simulink model "Task5_without_Scalar"  (R2023b)
settings: Solver=FixedStepAuto  StartTime=0.0  StopTime=300  FixedStep=.02  RelTol=1e-3
InitFcn:
  | run("Longitudinal_Autopilot.m")
values from neighbouring files (symbols this model uses):
  A_Long = [Xu                    Xw                        -w0                            -gravity*cos(theta0) ... (first row only)    [Longitudinal_Autopilot.m]
  B_Long = [Xde                         Xdth ... (first row only)    [Longitudinal_Autopilot.m]
  C_Long = eye(4)    [Longitudinal_Autopilot.m]
  D_Long = zeros(4,2)    [Longitudinal_Autopilot.m]
undefined symbols (not defined in the file or in its folder): sigbuilder_block, states_0, theta0, u0, w0
libraries: simulink_extras x28, cstblocks x21, slpidlib x5
settings Model: Creator=Saif Mohamed  LastModifiedBy=Saif Mohamed

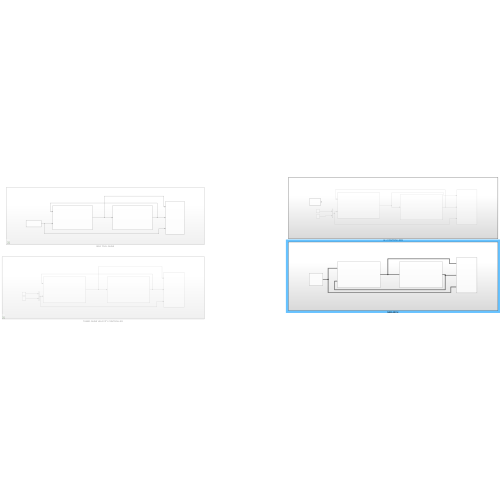
[thumbnail: Simulink's stored preview of the top-level diagram]
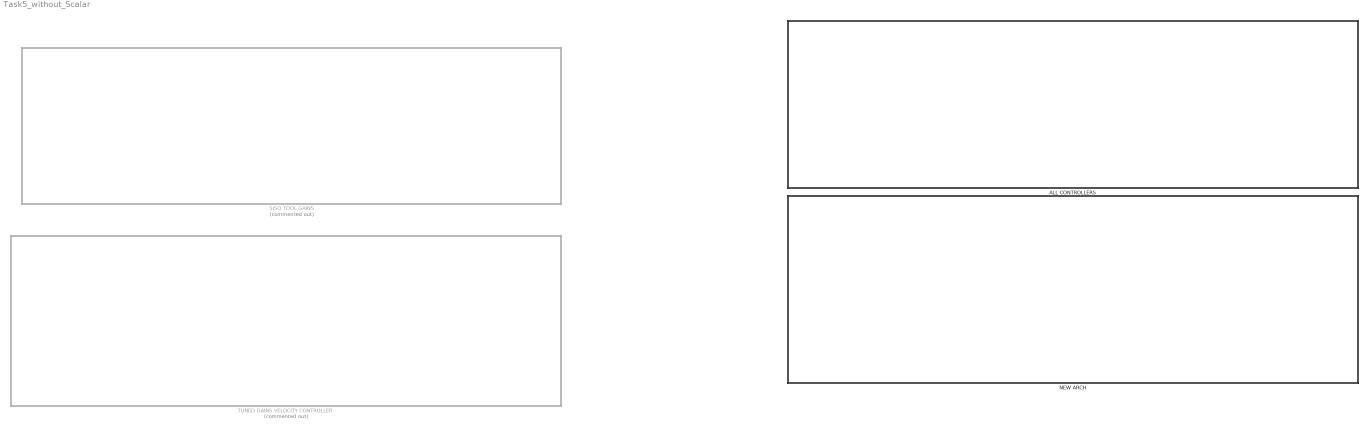
== system Task5_without_Scalar ==
  ALL CONTROLLERS : Subsystem
  "NEW ARCH " : Subsystem
  SISO TOOL GAINS : Subsystem  Commented=on
  "TUNED GAINS VELOCITY CONTROLLER " : Subsystem  Commented=on

== system Task5_without_Scalar/ALL CONTROLLERS ==
  Bus Creator1 : BusCreator  Commented=on  Inputs=2
  Constant2 : Constant  Commented=on  Value=100
  Constant3 : Constant  Commented=on  Value=20
  Display1 : Subsystem  Commented=on
  Longitudinal Model with height : Subsystem  Commented=on
  Signal Builder : Subsystem  Tag=STV Subsys  Commented=on  LoadFcn=sigbuilder_block('load');  StartFcn=sigbuilder_block('start');  StopFcn=sigbuilder_block('stop');  ClipboardFcn=sigbuilder_block('clipboard');  mask(Sigbuilder block){tuvar=[0:10]}
      mask help: Simulink:masks:SigbuilderBlock_MD
      mask init:
      | if ~strcmp(get_param(bdroot(gcbh),'SimulationStatus'),'stopped') tuvar = sigbuilder_block('maskInit'); end
      settings: CopyFcn=sigbuilder_block('copy');  DeleteFcn=sigbuilder_block('delete');  ModelCloseFcn=sigbuilder_block('modelClose');  PreSaveFcn=sigbuilder_block('preSave');  PauseFcn=sigbuilder_block('pause');  ContinueFcn=sigbuilder_block('continue');  NameChangeFcn=sigbuilder_block('namechange');  OpenFcn=sigbuilder_block('open',[5.4 36 1141.2 516.6 ]);  CloseFcn=sigbuilder_block('close');
      mask Display: plot(0, 0, 100, 100,[2, 2, 32, 32, 2], [68, 8, 8, 68, 68],[32, 2], [38, 38], [32, 19, 2],[53, 60, 44], [32, 17, 17, 2],[16, 16, 31, 31]);txt = getActiveGroup(gcbh);text(2, 100, txt,'verticalAlignment', 'top');
  State Space Model1 : Subsystem  Commented=on
  wires:
  Constant2/1 -> Bus Creator1/1  "height_comm"
  Longitudinal Model with height/1(Control_Actions) -> State Space Model1/1(Control_Actions), Display1/1(Control_Actions)
  Constant3/1 -> Bus Creator1/2  "u_command"
  State Space Model1/1(deltas) -> Display1/2(deltas), Longitudinal Model with height/1(deltas)
  Bus Creator1/1 -> Longitudinal Model with height/2(Command), Display1/3(Command)

== system Task5_without_Scalar/NEW ARCH  ==
  Display2 : Subsystem
  Longitudinal Model1 : Subsystem
  State Space Model2 : Subsystem
  Subsystem : Subsystem
  wires:
  Longitudinal Model1/1(Control_Actions) -> Display2/1(Control_Actions), State Space Model2/1(Control_Actions)
  Subsystem/1(Commands) -> Longitudinal Model1/1(Commands), Display2/3(Commands)
  State Space Model2/1(states) -> Longitudinal Model1/2(states), Display2/2(states)

== system Task5_without_Scalar/SISO TOOL GAINS ==
  Display3 : Subsystem
  Longitudinal Model2 : Subsystem
  State Space Model3 : Subsystem
  Subsystem : Subsystem
  wires:
  Longitudinal Model2/1(Control_Actions) -> Display3/1(Control_Actions), State Space Model3/1(Control_Actions)
  State Space Model3/1(deltas) -> Longitudinal Model2/1(deltas), Display3/2(deltas)
  Subsystem/1(Commands) -> Display3/3(Command), Longitudinal Model2/2(Commands)

== system Task5_without_Scalar/TUNED GAINS VELOCITY CONTROLLER  ==
  Bus Creator : BusCreator  Commented=on  Inputs=2
  Constant : Constant  Commented=on
  Constant1 : Constant  Commented=on  Value=10
  Display : Subsystem  Commented=on
  Longitudinal Model : Subsystem  Commented=on
  State Space Model : Subsystem  Commented=on
  wires:
  State Space Model/1(deltas) -> Longitudinal Model/1(deltas), Display/2(deltas)
  Longitudinal Model/1(Control_Actions) -> Display/1(Control_Actions), State Space Model/1(Control_Actions)
  Bus Creator/1 -> Display/3(Command), Longitudinal Model/2(Command)
  Constant/1 -> Bus Creator/1  "theta_command"
  Constant1/1 -> Bus Creator/2  "u_command"

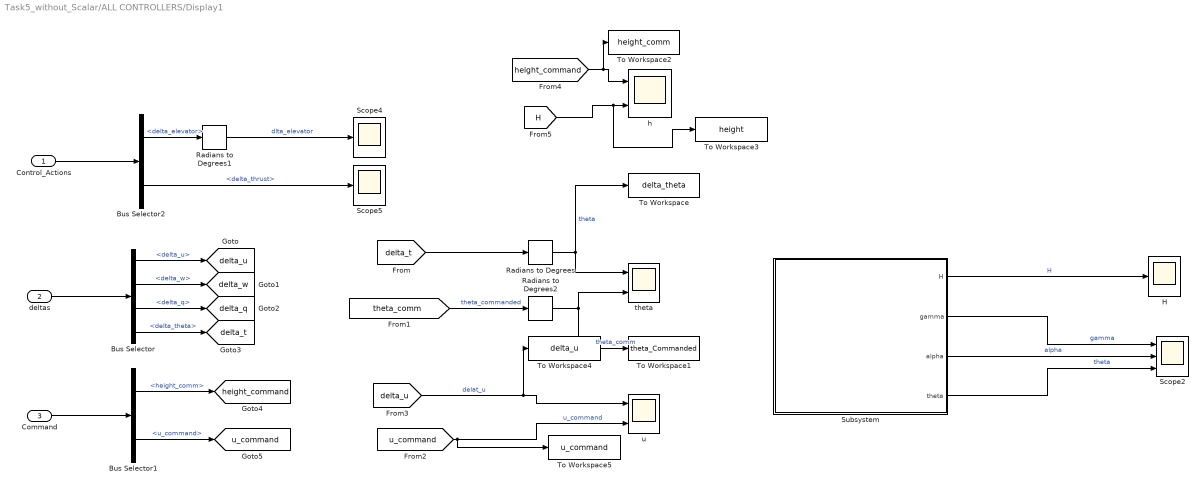
== system Task5_without_Scalar/ALL CONTROLLERS/Display1 ==
  Control_Actions : Inport
  deltas : Inport  Port=2
  Command : Inport  Port=3
  Bus Selector : BusSelector  OutputSignals=delta_u,delta_w,delta_q,delta_theta
  Bus Selector1 : BusSelector  OutputSignals=height_comm,u_command
  Bus Selector2 : BusSelector  OutputSignals=delta_elevator,delta_thrust
  H : Scope
  Radians to Degrees : simulink_extras/Transformations/Radians to Degrees
  Radians to Degrees1 : simulink_extras/Transformations/Radians to Degrees
  Radians to Degrees2 : simulink_extras/Transformations/Radians to Degrees
  Scope2 : Scope  NumInputPorts=3
  Scope4 : Scope
  Scope5 : Scope
  Subsystem : Subsystem
  To Workspace : ToWorkspace  VariableName=delta_theta  SampleTime=-1
  To Workspace1 : ToWorkspace  VariableName=theta_Commanded  SampleTime=-1
  To Workspace2 : ToWorkspace  VariableName=height_comm  SampleTime=-1
  To Workspace3 : ToWorkspace  VariableName=height  SampleTime=-1
  To Workspace4 : ToWorkspace  VariableName=delta_u  SampleTime=-1
  To Workspace5 : ToWorkspace  VariableName=u_command  SampleTime=-1
  h : Scope  NumInputPorts=2
  theta : Scope  NumInputPorts=2
  u : Scope  NumInputPorts=2
  tag scope: delta_q=global, delta_t=global, delta_u=global, delta_w=global, height_command=global, u_command=global
  wires:
  Radians to Degrees1/1 -> Scope4/1  "dlta_elevator"
  Bus Selector2/2 -> Scope5/1  "<delta_thrust>"
  Bus Selector2/1 -> Radians to Degrees1/1  "<delta_elevator>"
  Control_Actions/1 -> Bus Selector2/1
  [delta_u] -> To Workspace4/1, u/1  "delat_u"
  [u_command] -> To Workspace5/1, u/2  "u_command"
  Bus Selector1/2 -> [u_command]  "<u_command>"
  Bus Selector1/1 -> [height_command]  "<height_comm>"
  Command/1 -> Bus Selector1/1
  Subsystem/4(theta) -> Scope2/3  "theta"
  Subsystem/2(gamma) -> Scope2/1  "gamma"
  Subsystem/3(alpha) -> Scope2/2  "alpha"
  Subsystem/1(H) -> H/1  "H"
  [theta_comm] -> Radians to Degrees2/1  "theta_commanded"
  Radians to Degrees/1 -> theta/1, To Workspace/1  "theta"
  [delta_t] -> Radians to Degrees/1
  Bus Selector/4 -> [delta_t]  "<delta_theta>"
  Bus Selector/3 -> [delta_q]  "<delta_q>"
  Bus Selector/2 -> [delta_w]  "<delta_w>"
  Bus Selector/1 -> [delta_u]  "<delta_u>"
  deltas/1 -> Bus Selector/1
  [height_command] -> To Workspace2/1, h/1
  [H] -> To Workspace3/1, h/2
  Radians to Degrees2/1 -> theta/2, To Workspace1/1  "theta_comm"

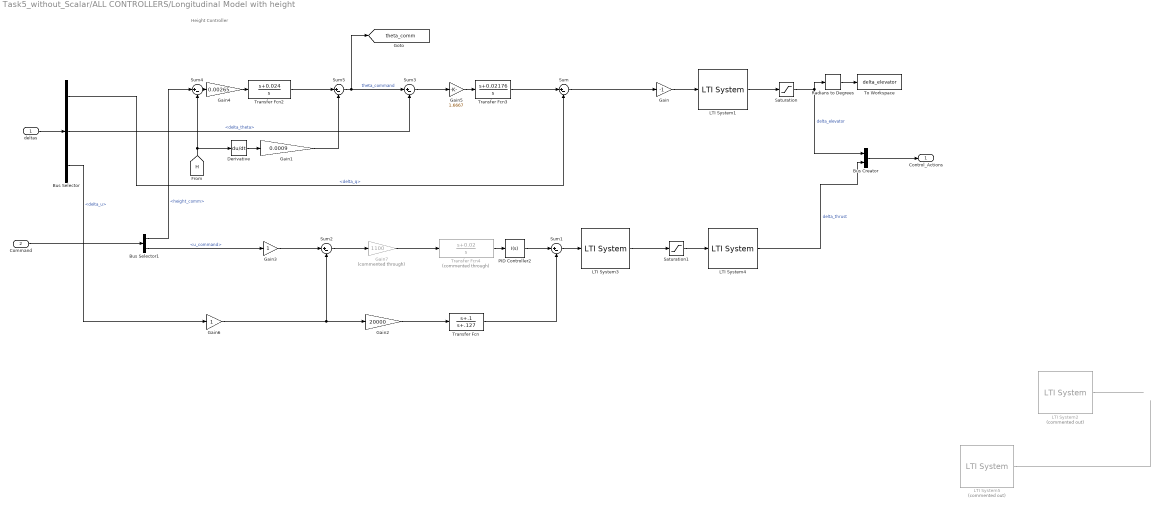
== system Task5_without_Scalar/ALL CONTROLLERS/Longitudinal Model with height ==
  note: Height Controller
  deltas : Inport
  Command : Inport  Port=2
  Bus Creator : BusCreator  Inputs=2
  Bus Selector : BusSelector  OutputSignals=delta_q,delta_theta,delta_u
  Bus Selector1 : BusSelector  OutputSignals=height_comm,u_command
  Derivative : Derivative
  Gain : Gain  Gain=-1
  Gain1 : Gain  Gain=0.0009
  Gain2 : Gain  Gain=20000
  Gain3 : Gain
  Gain4 : Gain  Gain=0.00265
  Gain5 : Gain  Gain=1.6667
  Gain6 : Gain
  Gain7 : Gain  Commented=through  Gain=1100
  LTI System1 : cstblocks/LTI System  sys=servo  IC=[]  PadeOrder=0
  LTI System2 : cstblocks/LTI System  Commented=on  sys=PI_U  IC=[]  PadeOrder=0
  LTI System3 : cstblocks/LTI System  sys=servo  IC=[]  PadeOrder=0
  LTI System4 : cstblocks/LTI System  sys=Engine_Lag  IC=[]  PadeOrder=0
  LTI System5 : cstblocks/LTI System  Commented=on  sys=Compensator  IC=[]  PadeOrder=0
  PID Controller2 : slpidlib/PID Controller  Controller=I  Form=Parallel  TimeDomain=Continuous-time  UseExternalTs=off  SampleTime=-1  IntegratorMethod=Forward Euler  FilterMethod=Forward Euler  ControllerParametersSource=internal  P=25000  I=150  UseKiTs=off  D=45918.9077381397  N=24.6739321802593  UseFilter=on  TunerSelectOption=Transfer Function Based (PID Tuner App)  InitialConditionSource=internal  InitialConditionForIntegrator=0  InitialConditionForFilter=0  DifferentiatorICPrevScaledInput=0  ExternalReset=none  TrackingMode=off  Kt=1  LimitOutput=off  SatLimitsSource=internal  UpperSaturationLimit=inf  LowerSaturationLimit=-inf  LinearizeAsGain=on  AntiWindupMode=none  Kb=1  LimitIntegrator=off  UpperIntegratorSaturationLimit=inf  LowerIntegratorSaturationLimit=-inf  POutMin=[]  POutMax=[]  IOutMin=[]  IOutMax=[]  DOutMin=[]  DOutMax=[]  NOutMin=[]  NOutMax=[]  SumOutMin=[]  SumOutMax=[]  SaturationOutMin=[]  SaturationOutMax=[]  PParamMin=[]  PParamMax=[]  IParamMin=[]  IParamMax=[]  DParamMin=[]  DParamMax=[]  NParamMin=[]  NParamMax=[]  KbParamMin=[]  KbParamMax=[]  KtParamMin=[]  KtParamMax=[]  KbOutMin=[]  KbOutMax=[]  KtOutMin=[]  KtOutMax=[]  IntegratorOutMin=[]  IntegratorOutMax=[]  FilterOutMin=[]  FilterOutMax=[]  SumI1OutMin=[]  SumI1OutMax=[]  SumI2OutMin=[]  SumI2OutMax=[]  SumI3OutMin=[]  SumI3OutMax=[]  SumI4OutMin=[]  SumI4OutMax=[]  SumDOutMin=[]  SumDOutMax=[]  DifferentiatorOutMin=[]  DifferentiatorOutMax=[]  FilterDiffOutCoefMin=[]  FilterDiffOutCoefMax=[]  ReciprocalOutMin=[]  ReciprocalOutMax=[]  SumDenOutMin=[]  SumDenOutMax=[]  SumNumOutMin=[]  SumNumOutMax=[]  DivideOutMin=[]  DivideOutMax=[]  UdiffTsProdOutMin=[]  UdiffTsProdOutMax=[]  NTsProdOutMin=[]  NTsProdOutMax=[]  UintegralTsProdOutMin=[]  UintegralTsProdOutMax=[]  UngainTsProdOutMin=[]  UngainTsProdOutMax=[]  ClampingZeroOutDataTypeStr=Inherit: Inherit via back propagation  ClampingZeroOutMin=[]  ClampingZeroOutMax=[]  FilterDenConstantOutDataTypeStr=Inherit: Inherit via back propagation  FilterDenConstantOutMin=[]  FilterDenConstantOutMax=[]  PCopyOutDataTypeStr=Inherit: Inherit via back propagation  PCopyOutMin=[]  PCopyOutMax=[]  NCopyOutDataTypeStr=Inherit: Inherit via back propagation  NCopyOutMin=[]  NCopyOutMax=[]  IntegratorContinuousStateAttributes=''  IntegratorStateMustResolveToSignalObject=off  IntegratorRTWStateStorageClass=Auto  FilterContinuousStateAttributes=''  FilterStateMustResolveToSignalObject=off  FilterRTWStateStorageClass=Auto  ParallelPVariant=Disabled  IdealPVariant=Disabled  IVariant=InternalParameters  DVariant=Disabled  IntegratorVariant=Continuous  SatVariant=Disabled  AWVariant=Passthrough  PCopyVariant=Disabled  TRVariant=Disabled  FdbkBlocksVariant=Forward  IdealPFdbkVariant=Disabled  SatFdbkVariant=Disabled  DerivativeFilterVariant=Disabled  NVariant=Disabled  NCopyVariant=Disabled_SignalSpec  FilterICVariant=Disabled  IntegratorICVariant=InternalICs  ExternalResetVariant=Disabled  TRSumVariant=Passthrough  SumFdbkVariant=Disabled  SumVariant=Passthrough_I  TsampFilterVariant=InternalTs  TsampNgainVariant=Passthrough  TsampIntegralVariant=Disabled_SignalSpec  ExternalSaturationOutDataTypeStr=Inherit: Same as second input
  Radians to Degrees : simulink_extras/Transformations/Radians to Degrees
  Saturation : Saturate  UpperLimit=deg2rad(25)  LowerLimit=deg2rad(-25)
  Saturation1 : Saturate  UpperLimit=65369  LowerLimit=-269369.84
  Sum{,1..5} (6 alike) : Sum  Inputs=|+-
  To Workspace : ToWorkspace  VariableName=delta_elevator  SampleTime=-1
  Transfer Fcn : TransferFcn  Numerator=[1 .1]  Denominator=[1 .127]
  Transfer Fcn2 : TransferFcn  Numerator=[1 0.024]  Denominator=[1 0]
  Transfer Fcn3 : TransferFcn  Numerator=[1 0.02176]  Denominator=[1 0]
  Transfer Fcn4 : TransferFcn  Commented=through  Numerator=[1 0.02]  Denominator=[1 0]
  Control_Actions : Outport
  tag scope: theta_comm=global
  wires:
  Transfer Fcn3/1 -> Sum/1
  Radians to Degrees/1 -> To Workspace/1
  Bus Creator/1 -> Control_Actions/1
  Saturation/1 -> Radians to Degrees/1, Bus Creator/1  "delta_elevator"
  LTI System1/1 -> Saturation/1
  Gain/1 -> LTI System1/1
  Sum/1 -> Gain/1
  Bus Selector/1 -> Sum/2  "<delta_q>"
  Bus Selector/2 -> Sum3/2  "<delta_theta>"
  Command/1 -> Bus Selector1/1
  deltas/1 -> Bus Selector/1
  Bus Selector1/1 -> Sum4/1  "<height_comm>"
  Sum5/1 -> [theta_comm], Sum3/1  "theta_command"
  Derivative/1 -> Gain1/1
  Gain1/1 -> Sum5/2
  Bus Selector1/2 -> Gain3/1  "<u_command>"
  LTI System4/1 -> Bus Creator/2  "delta_thrust"
  Saturation1/1 -> LTI System4/1
  Bus Selector/3 -> Gain6/1  "<delta_u>"
  LTI System3/1 -> Saturation1/1
  Gain5/1 -> Transfer Fcn3/1
  Sum3/1 -> Gain5/1
  Gain6/1 -> Sum2/2, Gain2/1
  Gain4/1 -> Transfer Fcn2/1
  Sum4/1 -> Gain4/1
  Gain3/1 -> Sum2/1
  LTI System2/1 -> ?
  LTI System5/1 -> ?
  ? -> LTI System5/1
  ? -> LTI System2/1
  Transfer Fcn/1 -> Sum1/2
  Sum2/1 -> Gain7/1
  Transfer Fcn4/1 -> PID Controller2/1
  Gain7/1 -> Transfer Fcn4/1
  Gain2/1 -> Transfer Fcn/1
  Sum1/1 -> LTI System3/1
  PID Controller2/1 -> Sum1/1
  Transfer Fcn2/1 -> Sum5/1
  [H] -> Sum4/2, Derivative/1

== system Task5_without_Scalar/ALL CONTROLLERS/Signal Builder ==
  Demux : Demux  Tag=STV Demux  Outputs=1
      settings: DisplayOption=none
  FromWs : FromWorkspace  Tag=STV FromWs  VariableName=tuvar
      SigBuilderData=|
      | common.afterFinalStr = 'Extrapolate'
      | common.sampleTime = 0
      | dataSet.timeRange = [0 1000]
      | dataSet.name = 'log_0_2021-4-14-21-54-39_vehicl'
      | sbobj.Name = 'Signal Builder'
      | sbobj.Groups.Name = 'log_0_2021-4-14-21-54-39_vehicl'
      | sbobj.Groups.Signals.Name = 'Signal 1'
      | sbobj.Groups.Signals.XData = [0 50 100 150 200 250 300 350 400 450 500 550 600 650 700 750 800 850 900 950 1000]
      | sbobj.Groups.Signals.YData = [0 940 1260 1540 1100 1400 1700 2000 2300 2600 2900 3200 3500 3800 4100 4400 6000 6000 6000 6000 6000]
      | sbobj.Groups.TimeRange = [0 1000]
  Signal 1 : Outport  Tag=STV Outport
  wires:
  FromWs/1 -> Demux/1
  Demux/1 -> Signal 1/1

== system Task5_without_Scalar/ALL CONTROLLERS/State Space Model1 ==
  Control_Actions : Inport
  Bus Creator1 : BusCreator  Inputs=4
  Bus Selector : BusSelector  OutputSignals=delta_elevator,delta_thrust
  Demux : Demux
  Gain : Gain  Gain=0
  Manual Switch : ManualSwitch
  Mux : Mux  Inputs=2
  State-Space : StateSpace  A=A_Long  B=B_Long  C=C_Long  D=D_Long  InitialCondition=0
  deltas : Outport
  wires:
  Bus Selector/2 -> Manual Switch/1, Gain/1  "<delta_thrust>"
  Bus Selector/1 -> Mux/1  "<delta_elevator>"
  Control_Actions/1 -> Bus Selector/1
  Gain/1 -> Manual Switch/2
  Manual Switch/1 -> Mux/2
  Demux/4 -> Bus Creator1/4  "delta_theta"
  State-Space/1 -> Demux/1
  Bus Creator1/1 -> deltas/1
  Demux/1 -> Bus Creator1/1  "delta_u"
  Demux/2 -> Bus Creator1/2  "delta_w"
  Mux/1 -> State-Space/1
  Demux/3 -> Bus Creator1/3  "delta_q"

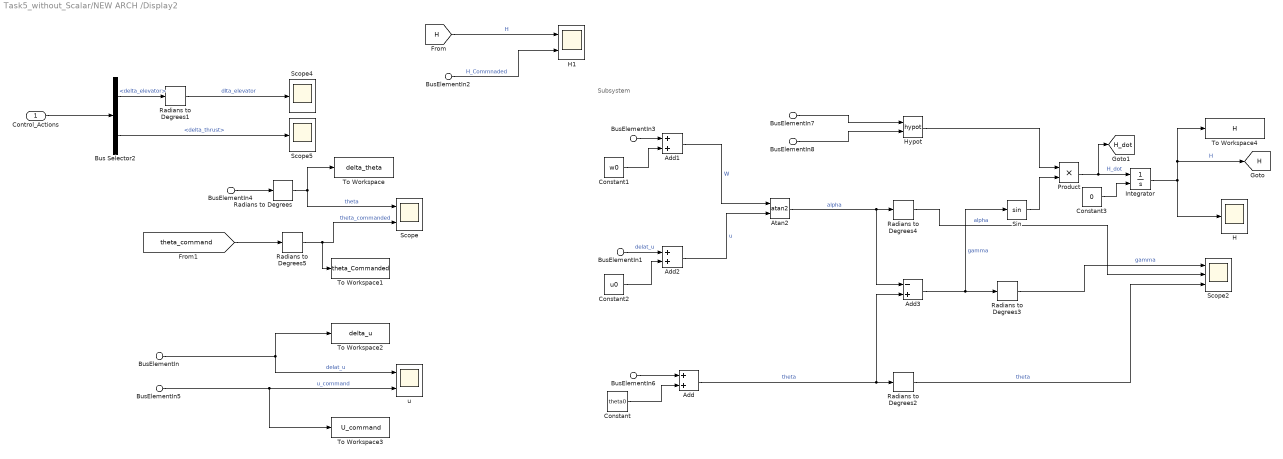
== system Task5_without_Scalar/NEW ARCH /Display2 ==
  note: Subsystem
  Control_Actions : Inport
  BusElementIn : Inport  Port=2  PortName=states  Element=States.delta_u
  BusElementIn1 : Inport  Port=2  PortName=states  Element=States.delta_u
  BusElementIn7 : Inport  Port=2  PortName=states  Element=States.delta_u
  BusElementIn4 : Inport  Port=2  PortName=states  Element=States.delta_theta
  BusElementIn6 : Inport  Port=2  PortName=states  Element=States.delta_theta
  BusElementIn3 : Inport  Port=2  PortName=states  Element=States.delta_w
  BusElementIn8 : Inport  Port=2  PortName=states  Element=States.delta_w
  BusElementIn5 : Inport  Port=3  PortName=Commands  Element=Command.u_command
  BusElementIn2 : Inport  Port=3  PortName=Commands  Element=Command.H_dot_command
  Add : Sum
  Add1 : Sum
  Add2 : Sum
  Add3 : Sum  Inputs=-+
  Atan2 : Trigonometry  Operator=atan2
  Bus Selector2 : BusSelector  OutputSignals=delta_elevator,delta_thrust
  Constant : Constant  Value=theta0
  Constant1 : Constant  Value=w0
  Constant2 : Constant  Value=u0
  Constant3 : Constant  Value=0
  H : Scope
  H1 : Scope  NumInputPorts=2
  Hypot : Math  Operator=hypot
  Integrator : Integrator  InitialConditionSource=external  InitialCondition=-states_0(12)
  Product : Product
  Radians to Degrees{,1..5} (6 alike) : simulink_extras/Transformations/Radians to Degrees
  Scope : Scope  NumInputPorts=2
  Scope2 : Scope  NumInputPorts=3
  Scope4 : Scope
  Scope5 : Scope
  Sin : Trigonometry
  To Workspace : ToWorkspace  VariableName=delta_theta  SampleTime=-1
  To Workspace1 : ToWorkspace  VariableName=theta_Commanded  SampleTime=-1
  To Workspace2 : ToWorkspace  VariableName=delta_u  SampleTime=-1
  To Workspace3 : ToWorkspace  VariableName=U_command  SampleTime=-1
  To Workspace4 : ToWorkspace  VariableName=H  SampleTime=-1
  u : Scope  NumInputPorts=2
  tag scope: H=global, H_dot=global
  wires:
  Radians to Degrees1/1 -> Scope4/1  "dlta_elevator"
  Bus Selector2/2 -> Scope5/1  "<delta_thrust>"
  Bus Selector2/1 -> Radians to Degrees1/1  "<delta_elevator>"
  Control_Actions/1 -> Bus Selector2/1
  BusElementIn/1 -> To Workspace2/1, u/1  "delat_u"
  BusElementIn5/1 -> To Workspace3/1, u/2  "u_command"
  Radians to Degrees2/1 -> Scope2/3  "theta"
  Radians to Degrees3/1 -> Scope2/1  "gamma"
  Radians to Degrees4/1 -> Scope2/2  "alpha"
  Radians to Degrees/1 -> Scope/1, To Workspace/1  "theta"
  BusElementIn4/1 -> Radians to Degrees/1
  BusElementIn8/1 -> Hypot/2
  Integrator/1 -> [H], To Workspace4/1, H/1  "H"
  BusElementIn6/1 -> Add/1
  Add/1 -> Add3/2, Radians to Degrees2/1  "theta"
  BusElementIn7/1 -> Hypot/1
  Constant1/1 -> Add1/2
  Sin/1 -> Product/2
  Constant2/1 -> Add2/2
  Constant/1 -> Add/2
  Add3/1 -> Sin/1, Radians to Degrees3/1  "gamma"
  Product/1 -> [H_dot], Integrator/1  "H_dot"
  Add2/1 -> Atan2/2  "u"
  Atan2/1 -> Radians to Degrees4/1, Add3/1  "alpha"
  Hypot/1 -> Product/1
  Add1/1 -> Atan2/1  "W"
  BusElementIn1/1 -> Add2/1  "delat_u"
  BusElementIn3/1 -> Add1/1
  [theta_command] -> Radians to Degrees5/1
  Radians to Degrees5/1 -> To Workspace1/1, Scope/2  "theta_commanded"
  [H] -> H1/1  "H"
  BusElementIn2/1 -> H1/2  "H_Commnaded"
  Constant3/1 -> Integrator/2

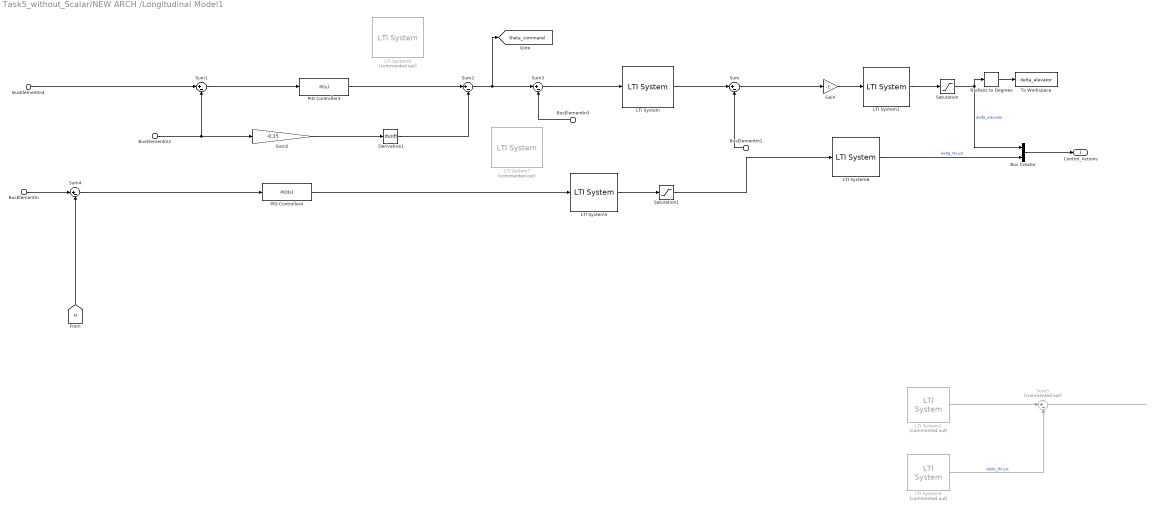
== system Task5_without_Scalar/NEW ARCH /Longitudinal Model1 ==
  BusElementIn : Inport  PortName=Commands  Element=Command.H_dot_command
  BusElementIn4 : Inport  PortName=Commands  Element=Command.u_command
  BusElementIn2 : Inport  Port=2  PortName=states  Element=States.delta_u
  BusElementIn1 : Inport  Port=2  PortName=states  Element=States.delta_q
  BusElementIn3 : Inport  Port=2  PortName=states  Element=States.delta_theta
  Bus Creator : BusCreator  Inputs=2
  Derivative1 : Derivative
  Gain : Gain  Gain=-1
  Gain2 : Gain  Gain=-0.15
  LTI System : cstblocks/LTI System  sys=PI_Pitch  IC=[]  PadeOrder=0
  LTI System1 : cstblocks/LTI System  sys=servo  IC=[]  PadeOrder=0
  LTI System2 : cstblocks/LTI System  Commented=on  sys=C1_H_dot  IC=[]  PadeOrder=0
  LTI System4 : cstblocks/LTI System  Commented=on  sys=C2_H_dot  IC=[]  PadeOrder=0
  LTI System5 : cstblocks/LTI System  sys=servo  IC=[]  PadeOrder=0
  LTI System6 : cstblocks/LTI System  sys=Engine_Lag  IC=[]  PadeOrder=0
  LTI System7 : cstblocks/LTI System  Commented=on  sys=Compenstor_U_Theta  IC=[]  PadeOrder=0
  LTI System8 : cstblocks/LTI System  Commented=on  sys=PI_U_theta  IC=[]  PadeOrder=0
  PID Controller3 : slpidlib/PID Controller  Controller=PI  Form=Parallel  TimeDomain=Continuous-time  UseExternalTs=off  SampleTime=-1  IntegratorMethod=Forward Euler  FilterMethod=Forward Euler  ControllerParametersSource=internal  P=-0.07  I=-0.0055  UseKiTs=off  D=-0.0999  N=1.3873123315198  UseFilter=on  TunerSelectOption=Transfer Function Based (PID Tuner App)  InitialConditionSource=internal  InitialConditionForIntegrator=0  InitialConditionForFilter=0  DifferentiatorICPrevScaledInput=0  ExternalReset=none  TrackingMode=off  Kt=1  LimitOutput=off  SatLimitsSource=internal  UpperSaturationLimit=inf  LowerSaturationLimit=-inf  LinearizeAsGain=on  AntiWindupMode=none  Kb=1  LimitIntegrator=off  UpperIntegratorSaturationLimit=inf  LowerIntegratorSaturationLimit=-inf  POutMin=[]  POutMax=[]  IOutMin=[]  IOutMax=[]  DOutMin=[]  DOutMax=[]  NOutMin=[]  NOutMax=[]  SumOutMin=[]  SumOutMax=[]  SaturationOutMin=[]  SaturationOutMax=[]  PParamMin=[]  PParamMax=[]  IParamMin=[]  IParamMax=[]  DParamMin=[]  DParamMax=[]  NParamMin=[]  NParamMax=[]  KbParamMin=[]  KbParamMax=[]  KtParamMin=[]  KtParamMax=[]  KbOutMin=[]  KbOutMax=[]  KtOutMin=[]  KtOutMax=[]  IntegratorOutMin=[]  IntegratorOutMax=[]  FilterOutMin=[]  FilterOutMax=[]  SumI1OutMin=[]  SumI1OutMax=[]  SumI2OutMin=[]  SumI2OutMax=[]  SumI3OutMin=[]  SumI3OutMax=[]  SumI4OutMin=[]  SumI4OutMax=[]  SumDOutMin=[]  SumDOutMax=[]  DifferentiatorOutMin=[]  DifferentiatorOutMax=[]  FilterDiffOutCoefMin=[]  FilterDiffOutCoefMax=[]  ReciprocalOutMin=[]  ReciprocalOutMax=[]  SumDenOutMin=[]  SumDenOutMax=[]  SumNumOutMin=[]  SumNumOutMax=[]  DivideOutMin=[]  DivideOutMax=[]  UdiffTsProdOutMin=[]  UdiffTsProdOutMax=[]  NTsProdOutMin=[]  NTsProdOutMax=[]  UintegralTsProdOutMin=[]  UintegralTsProdOutMax=[]  UngainTsProdOutMin=[]  UngainTsProdOutMax=[]  ClampingZeroOutDataTypeStr=Inherit: Inherit via back propagation  ClampingZeroOutMin=[]  ClampingZeroOutMax=[]  FilterDenConstantOutDataTypeStr=Inherit: Inherit via back propagation  FilterDenConstantOutMin=[]  FilterDenConstantOutMax=[]  PCopyOutDataTypeStr=Inherit: Inherit via back propagation  PCopyOutMin=[]  PCopyOutMax=[]  NCopyOutDataTypeStr=Inherit: Inherit via back propagation  NCopyOutMin=[]  NCopyOutMax=[]  IntegratorContinuousStateAttributes=''  IntegratorStateMustResolveToSignalObject=off  IntegratorRTWStateStorageClass=Auto  FilterContinuousStateAttributes=''  FilterStateMustResolveToSignalObject=off  FilterRTWStateStorageClass=Auto  ParallelPVariant=InternalParameters  IdealPVariant=Disabled  IVariant=InternalParameters  DVariant=Disabled  IntegratorVariant=Continuous  SatVariant=Disabled  AWVariant=Passthrough  PCopyVariant=Disabled  TRVariant=Disabled  FdbkBlocksVariant=Forward  IdealPFdbkVariant=Disabled  SatFdbkVariant=Disabled  DerivativeFilterVariant=Disabled  NVariant=Disabled  NCopyVariant=Disabled_SignalSpec  FilterICVariant=Disabled  IntegratorICVariant=InternalICs  ExternalResetVariant=Disabled  TRSumVariant=Passthrough  SumFdbkVariant=Disabled  SumVariant=Sum_PI  TsampFilterVariant=InternalTs  TsampNgainVariant=Passthrough  TsampIntegralVariant=Disabled_SignalSpec  ExternalSaturationOutDataTypeStr=Inherit: Same as second input
  PID Controller4 : slpidlib/PID Controller  Controller=PID  Form=Parallel  TimeDomain=Continuous-time  UseExternalTs=off  SampleTime=-1  IntegratorMethod=Forward Euler  FilterMethod=Forward Euler  ControllerParametersSource=internal  P=9500  I=0.5  UseKiTs=off  D=25000  N=100  UseFilter=on  TunerSelectOption=Transfer Function Based (PID Tuner App)  InitialConditionSource=internal  InitialConditionForIntegrator=0  InitialConditionForFilter=0  DifferentiatorICPrevScaledInput=0  ExternalReset=none  TrackingMode=off  Kt=1  LimitOutput=off  SatLimitsSource=internal  UpperSaturationLimit=inf  LowerSaturationLimit=-inf  LinearizeAsGain=on  AntiWindupMode=none  Kb=1  LimitIntegrator=off  UpperIntegratorSaturationLimit=inf  LowerIntegratorSaturationLimit=-inf  POutMin=[]  POutMax=[]  IOutMin=[]  IOutMax=[]  DOutMin=[]  DOutMax=[]  NOutMin=[]  NOutMax=[]  SumOutMin=[]  SumOutMax=[]  SaturationOutMin=[]  SaturationOutMax=[]  PParamMin=[]  PParamMax=[]  IParamMin=[]  IParamMax=[]  DParamMin=[]  DParamMax=[]  NParamMin=[]  NParamMax=[]  KbParamMin=[]  KbParamMax=[]  KtParamMin=[]  KtParamMax=[]  KbOutMin=[]  KbOutMax=[]  KtOutMin=[]  KtOutMax=[]  IntegratorOutMin=[]  IntegratorOutMax=[]  FilterOutMin=[]  FilterOutMax=[]  SumI1OutMin=[]  SumI1OutMax=[]  SumI2OutMin=[]  SumI2OutMax=[]  SumI3OutMin=[]  SumI3OutMax=[]  SumI4OutMin=[]  SumI4OutMax=[]  SumDOutMin=[]  SumDOutMax=[]  DifferentiatorOutMin=[]  DifferentiatorOutMax=[]  FilterDiffOutCoefMin=[]  FilterDiffOutCoefMax=[]  ReciprocalOutMin=[]  ReciprocalOutMax=[]  SumDenOutMin=[]  SumDenOutMax=[]  SumNumOutMin=[]  SumNumOutMax=[]  DivideOutMin=[]  DivideOutMax=[]  UdiffTsProdOutMin=[]  UdiffTsProdOutMax=[]  NTsProdOutMin=[]  NTsProdOutMax=[]  UintegralTsProdOutMin=[]  UintegralTsProdOutMax=[]  UngainTsProdOutMin=[]  UngainTsProdOutMax=[]  ClampingZeroOutDataTypeStr=Inherit: Inherit via back propagation  ClampingZeroOutMin=[]  ClampingZeroOutMax=[]  FilterDenConstantOutDataTypeStr=Inherit: Inherit via back propagation  FilterDenConstantOutMin=[]  FilterDenConstantOutMax=[]  PCopyOutDataTypeStr=Inherit: Inherit via back propagation  PCopyOutMin=[]  PCopyOutMax=[]  NCopyOutDataTypeStr=Inherit: Inherit via back propagation  NCopyOutMin=[]  NCopyOutMax=[]  IntegratorContinuousStateAttributes=''  IntegratorStateMustResolveToSignalObject=off  IntegratorRTWStateStorageClass=Auto  FilterContinuousStateAttributes=''  FilterStateMustResolveToSignalObject=off  FilterRTWStateStorageClass=Auto  ParallelPVariant=InternalParameters  IdealPVariant=Disabled  IVariant=InternalParameters  DVariant=InternalParameters  IntegratorVariant=Continuous  SatVariant=Disabled  AWVariant=Passthrough  PCopyVariant=Disabled  TRVariant=Disabled  FdbkBlocksVariant=Forward  IdealPFdbkVariant=Disabled  SatFdbkVariant=Disabled  DerivativeFilterVariant=ContFilter  NVariant=InternalParameters  NCopyVariant=Disabled  FilterICVariant=InternalICsFilter  IntegratorICVariant=InternalICs  ExternalResetVariant=Disabled  TRSumVariant=Passthrough  SumFdbkVariant=Disabled  SumVariant=Sum_PID  TsampFilterVariant=InternalTs  TsampNgainVariant=Passthrough  TsampIntegralVariant=Disabled_SignalSpec  ExternalSaturationOutDataTypeStr=Inherit: Same as second input
  Radians to Degrees : simulink_extras/Transformations/Radians to Degrees
  Saturation : Saturate  UpperLimit=deg2rad(25)  LowerLimit=deg2rad(-25)
  Saturation1 : Saturate  UpperLimit=65369  LowerLimit=-269369.84
  Sum{,1..4} (5 alike) : Sum  Inputs=|+-
  Sum5 : Sum  Commented=on  Inputs=|+-
  To Workspace : ToWorkspace  VariableName=delta_elevator  SampleTime=-1
  Control_Actions : Outport
  tag scope: theta_command=global
  wires:
  Radians to Degrees/1 -> To Workspace/1
  Bus Creator/1 -> Control_Actions/1
  Saturation/1 -> Radians to Degrees/1, Bus Creator/1  "delta_elevator"
  LTI System1/1 -> Saturation/1
  Gain/1 -> LTI System1/1
  Sum/1 -> Gain/1
  LTI System/1 -> Sum/1
  Sum3/1 -> LTI System/1
  Derivative1/1 -> Sum2/2
  Sum1/1 -> PID Controller3/1
  BusElementIn2/1 -> Gain2/1, Sum1/2
  BusElementIn3/1 -> Sum3/2
  BusElementIn1/1 -> Sum/2
  BusElementIn4/1 -> Sum1/1
  BusElementIn/1 -> Sum4/1
  LTI System5/1 -> Saturation1/1
  LTI System6/1 -> Bus Creator/2  "delta_thrust"
  Saturation1/1 -> LTI System6/1
  LTI System4/1 -> Sum5/2  "delta_thrust"
  Sum5/1 -> ?
  ? -> LTI System4/1
  ? -> LTI System2/1
  LTI System2/1 -> Sum5/1
  [H] -> Sum4/2
  Sum4/1 -> PID Controller4/1
  Gain2/1 -> Derivative1/1
  PID Controller3/1 -> Sum2/1
  Sum2/1 -> [theta_command], Sum3/1
  PID Controller4/1 -> LTI System5/1

== system Task5_without_Scalar/NEW ARCH /State Space Model2 ==
  Control_Actions : Inport
  Bus Creator1 : BusCreator  Inputs=4
  Bus Selector : BusSelector  OutputSignals=delta_elevator,delta_thrust
  Demux : Demux
  Gain : Gain  Gain=0
  Manual Switch : ManualSwitch
  Mux : Mux  Inputs=2
  State-Space : StateSpace  A=A_Long  B=B_Long  C=C_Long  D=D_Long  InitialCondition=0
  Out Bus Element : Outport  PortName=states  Element=States
  wires:
  Bus Selector/2 -> Manual Switch/1, Gain/1  "<delta_thrust>"
  Bus Selector/1 -> Mux/1  "<delta_elevator>"
  Control_Actions/1 -> Bus Selector/1
  Gain/1 -> Manual Switch/2
  Manual Switch/1 -> Mux/2
  Demux/4 -> Bus Creator1/4  "delta_theta"
  State-Space/1 -> Demux/1
  Bus Creator1/1 -> Out Bus Element/1
  Demux/1 -> Bus Creator1/1  "delta_u"
  Demux/2 -> Bus Creator1/2  "delta_w"
  Mux/1 -> State-Space/1
  Demux/3 -> Bus Creator1/3  "delta_q"

== system Task5_without_Scalar/NEW ARCH /Subsystem ==
  Bus Creator2 : BusCreator  Inputs=2
  Constant4 : Constant  Value=100
  Constant5 : Constant  Value=15
  Out Bus Element : Outport  PortName=Commands  Element=Command
  wires:
  Constant5/1 -> Bus Creator2/2  "u_command"
  Bus Creator2/1 -> Out Bus Element/1
  Constant4/1 -> Bus Creator2/1  "H_dot_command"

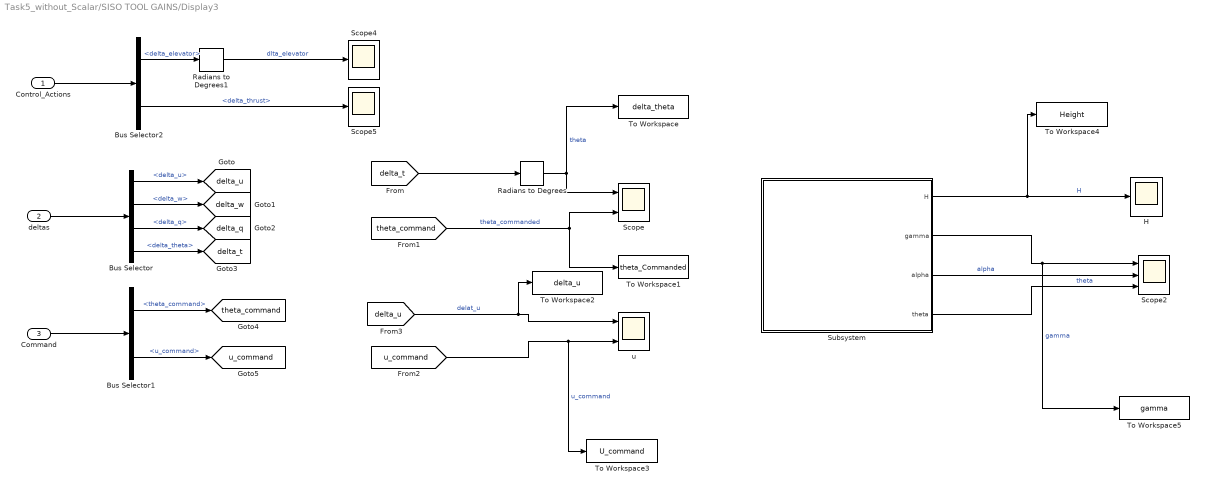
== system Task5_without_Scalar/SISO TOOL GAINS/Display3 ==
  Control_Actions : Inport
  deltas : Inport  Port=2
  Command : Inport  Port=3
  Bus Selector : BusSelector  OutputSignals=deltas.delta_u,deltas.delta_w,deltas.delta_q,deltas.delta_theta
  Bus Selector1 : BusSelector  OutputSignals=commands.theta_command,commands.u_command
  Bus Selector2 : BusSelector  OutputSignals=delta_elevator,delta_thrust
  H : Scope
  Radians to Degrees : simulink_extras/Transformations/Radians to Degrees
  Radians to Degrees1 : simulink_extras/Transformations/Radians to Degrees
  Scope : Scope  NumInputPorts=2
  Scope2 : Scope  NumInputPorts=3
  Scope4 : Scope
  Scope5 : Scope
  Subsystem : Subsystem
  To Workspace : ToWorkspace  VariableName=delta_theta  SampleTime=-1
  To Workspace1 : ToWorkspace  VariableName=theta_Commanded  SampleTime=-1
  To Workspace2 : ToWorkspace  VariableName=delta_u  SampleTime=-1
  To Workspace3 : ToWorkspace  VariableName=U_command  SampleTime=-1
  To Workspace4 : ToWorkspace  VariableName=Height  SampleTime=-1
  To Workspace5 : ToWorkspace  VariableName=gamma  SampleTime=-1
  u : Scope  NumInputPorts=2
  tag scope: delta_q=global, delta_t=global, delta_u=global, delta_w=global, theta_command=global, u_command=global
  wires:
  deltas/1 -> Bus Selector/1
  Bus Selector/1 -> [delta_u]  "<delta_u>"
  Bus Selector/2 -> [delta_w]  "<delta_w>"
  Bus Selector/3 -> [delta_q]  "<delta_q>"
  Bus Selector/4 -> [delta_t]  "<delta_theta>"
  [delta_t] -> Radians to Degrees/1
  Radians to Degrees/1 -> To Workspace/1, Scope/1  "theta"
  [theta_command] -> To Workspace1/1, Scope/2  "theta_commanded"
  Subsystem/1(H) -> To Workspace4/1, H/1  "H"
  Subsystem/3(alpha) -> Scope2/2  "alpha"
  Subsystem/2(gamma) -> To Workspace5/1, Scope2/1  "gamma"
  Subsystem/4(theta) -> Scope2/3  "theta"
  Command/1 -> Bus Selector1/1
  Bus Selector1/1 -> [theta_command]  "<theta_command>"
  Bus Selector1/2 -> [u_command]  "<u_command>"
  [u_command] -> To Workspace3/1, u/2  "u_command"
  [delta_u] -> To Workspace2/1, u/1  "delat_u"
  Control_Actions/1 -> Bus Selector2/1
  Bus Selector2/1 -> Radians to Degrees1/1  "<delta_elevator>"
  Bus Selector2/2 -> Scope5/1  "<delta_thrust>"
  Radians to Degrees1/1 -> Scope4/1  "dlta_elevator"

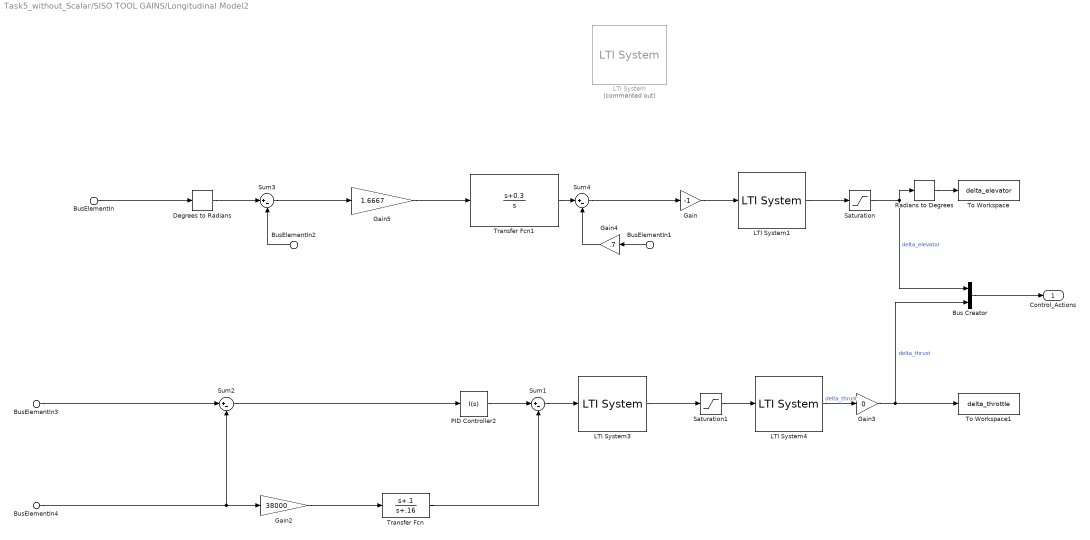
== system Task5_without_Scalar/SISO TOOL GAINS/Longitudinal Model2 ==
  BusElementIn1 : Inport  PortName=deltas  Element=deltas.delta_q
  BusElementIn2 : Inport  PortName=deltas  Element=deltas.delta_theta
  BusElementIn4 : Inport  PortName=deltas  Element=deltas.delta_u
  BusElementIn : Inport  Port=2  PortName=Commands  Element=commands.theta_command
  BusElementIn3 : Inport  Port=2  PortName=Commands  Element=commands.u_command
  Bus Creator : BusCreator  Inputs=2
  Degrees to Radians : simulink_extras/Transformations/Degrees to Radians
  Gain : Gain  Gain=-1
  Gain2 : Gain  Gain=38000
  Gain3 : Gain  Gain=0
  Gain4 : Gain  Gain=.7
  Gain5 : Gain  Gain=1.6667
  LTI System : cstblocks/LTI System  Commented=on  sys=PI_Pitch  IC=[]  PadeOrder=0
  LTI System1 : cstblocks/LTI System  sys=servo  IC=[]  PadeOrder=0
  LTI System3 : cstblocks/LTI System  sys=servo  IC=[]  PadeOrder=0
  LTI System4 : cstblocks/LTI System  sys=Engine_Lag  IC=[]  PadeOrder=0
  PID Controller2 : slpidlib/PID Controller  Controller=I  Form=Parallel  TimeDomain=Continuous-time  UseExternalTs=off  SampleTime=-1  IntegratorMethod=Forward Euler  FilterMethod=Forward Euler  ControllerParametersSource=internal  P=25000  I=1400  UseKiTs=off  D=45918.9077381397  N=24.6739321802593  UseFilter=on  TunerSelectOption=Transfer Function Based (PID Tuner App)  InitialConditionSource=internal  InitialConditionForIntegrator=0  InitialConditionForFilter=0  DifferentiatorICPrevScaledInput=0  ExternalReset=none  TrackingMode=off  Kt=1  LimitOutput=off  SatLimitsSource=internal  UpperSaturationLimit=inf  LowerSaturationLimit=-inf  LinearizeAsGain=on  AntiWindupMode=none  Kb=1  LimitIntegrator=off  UpperIntegratorSaturationLimit=inf  LowerIntegratorSaturationLimit=-inf  POutMin=[]  POutMax=[]  IOutMin=[]  IOutMax=[]  DOutMin=[]  DOutMax=[]  NOutMin=[]  NOutMax=[]  SumOutMin=[]  SumOutMax=[]  SaturationOutMin=[]  SaturationOutMax=[]  PParamMin=[]  PParamMax=[]  IParamMin=[]  IParamMax=[]  DParamMin=[]  DParamMax=[]  NParamMin=[]  NParamMax=[]  KbParamMin=[]  KbParamMax=[]  KtParamMin=[]  KtParamMax=[]  KbOutMin=[]  KbOutMax=[]  KtOutMin=[]  KtOutMax=[]  IntegratorOutMin=[]  IntegratorOutMax=[]  FilterOutMin=[]  FilterOutMax=[]  SumI1OutMin=[]  SumI1OutMax=[]  SumI2OutMin=[]  SumI2OutMax=[]  SumI3OutMin=[]  SumI3OutMax=[]  SumI4OutMin=[]  SumI4OutMax=[]  SumDOutMin=[]  SumDOutMax=[]  DifferentiatorOutMin=[]  DifferentiatorOutMax=[]  FilterDiffOutCoefMin=[]  FilterDiffOutCoefMax=[]  ReciprocalOutMin=[]  ReciprocalOutMax=[]  SumDenOutMin=[]  SumDenOutMax=[]  SumNumOutMin=[]  SumNumOutMax=[]  DivideOutMin=[]  DivideOutMax=[]  UdiffTsProdOutMin=[]  UdiffTsProdOutMax=[]  NTsProdOutMin=[]  NTsProdOutMax=[]  UintegralTsProdOutMin=[]  UintegralTsProdOutMax=[]  UngainTsProdOutMin=[]  UngainTsProdOutMax=[]  ClampingZeroOutDataTypeStr=Inherit: Inherit via back propagation  ClampingZeroOutMin=[]  ClampingZeroOutMax=[]  FilterDenConstantOutDataTypeStr=Inherit: Inherit via back propagation  FilterDenConstantOutMin=[]  FilterDenConstantOutMax=[]  PCopyOutDataTypeStr=Inherit: Inherit via back propagation  PCopyOutMin=[]  PCopyOutMax=[]  NCopyOutDataTypeStr=Inherit: Inherit via back propagation  NCopyOutMin=[]  NCopyOutMax=[]  IntegratorContinuousStateAttributes=''  IntegratorStateMustResolveToSignalObject=off  IntegratorRTWStateStorageClass=Auto  FilterContinuousStateAttributes=''  FilterStateMustResolveToSignalObject=off  FilterRTWStateStorageClass=Auto  ParallelPVariant=Disabled  IdealPVariant=Disabled  IVariant=InternalParameters  DVariant=Disabled  IntegratorVariant=Continuous  SatVariant=Disabled  AWVariant=Passthrough  PCopyVariant=Disabled  TRVariant=Disabled  FdbkBlocksVariant=Forward  IdealPFdbkVariant=Disabled  SatFdbkVariant=Disabled  DerivativeFilterVariant=Disabled  NVariant=Disabled  NCopyVariant=Disabled_SignalSpec  FilterICVariant=Disabled  IntegratorICVariant=InternalICs  ExternalResetVariant=Disabled  TRSumVariant=Passthrough  SumFdbkVariant=Disabled  SumVariant=Passthrough_I  TsampFilterVariant=InternalTs  TsampNgainVariant=Passthrough  TsampIntegralVariant=Disabled_SignalSpec  ExternalSaturationOutDataTypeStr=Inherit: Same as second input
  Radians to Degrees : simulink_extras/Transformations/Radians to Degrees
  Saturation : Saturate  UpperLimit=deg2rad(25)  LowerLimit=deg2rad(-25)
  Saturation1 : Saturate  UpperLimit=65369  LowerLimit=-269369.84
  Sum{1..4} (4 alike) : Sum  Inputs=|+-
  To Workspace : ToWorkspace  VariableName=delta_elevator  SampleTime=-1
  To Workspace1 : ToWorkspace  VariableName=delta_throttle  SampleTime=-1
  Transfer Fcn : TransferFcn  Numerator=[1 .1]  Denominator=[1 .16]
  Transfer Fcn1 : TransferFcn  Numerator=[1 0.3]  Denominator=[1 0]
  Control_Actions : Outport
  wires:
  BusElementIn/1 -> Degrees to Radians/1
  Degrees to Radians/1 -> Sum3/1
  Sum3/1 -> Gain5/1
  Gain/1 -> LTI System1/1
  LTI System1/1 -> Saturation/1
  Saturation/1 -> Bus Creator/1, Radians to Degrees/1  "delta_elevator"
  Bus Creator/1 -> Control_Actions/1
  Radians to Degrees/1 -> To Workspace/1
  Sum2/1 -> PID Controller2/1
  Sum1/1 -> LTI System3/1
  LTI System3/1 -> Saturation1/1
  Saturation1/1 -> LTI System4/1
  Transfer Fcn/1 -> Sum1/2
  LTI System4/1 -> Gain3/1  "delta_thrust"
  Gain2/1 -> Transfer Fcn/1
  PID Controller2/1 -> Sum1/1
  Gain3/1 -> Bus Creator/2, To Workspace1/1  "delta_thrust"
  BusElementIn2/1 -> Sum3/2
  BusElementIn1/1 -> Gain4/1
  BusElementIn3/1 -> Sum2/1
  BusElementIn4/1 -> Sum2/2, Gain2/1
  Gain4/1 -> Sum4/2
  Gain5/1 -> Transfer Fcn1/1
  Sum4/1 -> Gain/1
  Transfer Fcn1/1 -> Sum4/1

== system Task5_without_Scalar/SISO TOOL GAINS/State Space Model3 ==
  Control_Actions : Inport
  Bus Creator1 : BusCreator  Inputs=4
  Bus Selector : BusSelector  OutputSignals=delta_elevator,delta_thrust
  Demux : Demux
  Gain : Gain  Gain=0
  Manual Switch : ManualSwitch
  Mux : Mux  Inputs=2
  State-Space : StateSpace  A=A_Long  B=B_Long  C=C_Long  D=D_Long  InitialCondition=0
  Out Bus Element : Outport  PortName=deltas  Element=deltas
  wires:
  Demux/3 -> Bus Creator1/3  "delta_q"
  Mux/1 -> State-Space/1
  Demux/2 -> Bus Creator1/2  "delta_w"
  Demux/1 -> Bus Creator1/1  "delta_u"
  Bus Creator1/1 -> Out Bus Element/1
  State-Space/1 -> Demux/1
  Demux/4 -> Bus Creator1/4  "delta_theta"
  Manual Switch/1 -> Mux/2
  Gain/1 -> Manual Switch/2
  Control_Actions/1 -> Bus Selector/1
  Bus Selector/1 -> Mux/1  "<delta_elevator>"
  Bus Selector/2 -> Gain/1, Manual Switch/1  "<delta_thrust>"

== system Task5_without_Scalar/SISO TOOL GAINS/Subsystem ==
  Bus Creator2 : BusCreator  Inputs=2
  Constant4 : Constant  Value=15
  Constant5 : Constant  Value=10
  Out Bus Element : Outport  PortName=Commands  Element=commands
  wires:
  Constant4/1 -> Bus Creator2/1  "theta_command"
  Constant5/1 -> Bus Creator2/2  "u_command"
  Bus Creator2/1 -> Out Bus Element/1

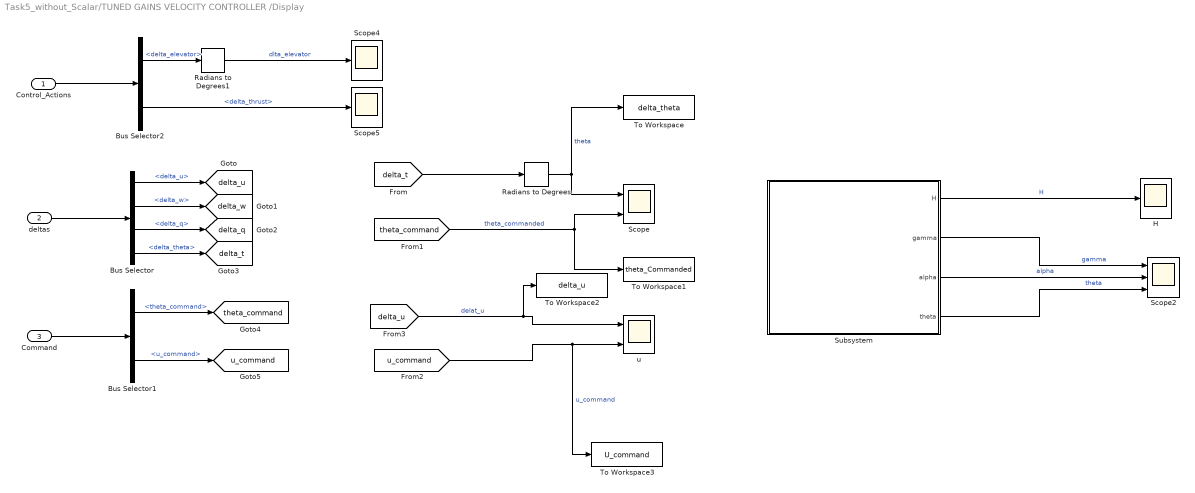
== system Task5_without_Scalar/TUNED GAINS VELOCITY CONTROLLER /Display ==
  Control_Actions : Inport
  deltas : Inport  Port=2
  Command : Inport  Port=3
  Bus Selector : BusSelector  OutputSignals=delta_u,delta_w,delta_q,delta_theta
  Bus Selector1 : BusSelector  OutputSignals=theta_command,u_command
  Bus Selector2 : BusSelector  OutputSignals=delta_elevator,delta_thrust
  H : Scope
  Radians to Degrees : simulink_extras/Transformations/Radians to Degrees
  Radians to Degrees1 : simulink_extras/Transformations/Radians to Degrees
  Scope : Scope  NumInputPorts=2
  Scope2 : Scope  NumInputPorts=3
  Scope4 : Scope
  Scope5 : Scope
  Subsystem : Subsystem
  To Workspace : ToWorkspace  VariableName=delta_theta  SampleTime=-1
  To Workspace1 : ToWorkspace  VariableName=theta_Commanded  SampleTime=-1
  To Workspace2 : ToWorkspace  VariableName=delta_u  SampleTime=-1
  To Workspace3 : ToWorkspace  VariableName=U_command  SampleTime=-1
  u : Scope  NumInputPorts=2
  tag scope: delta_q=global, delta_t=global, delta_u=global, delta_w=global, theta_command=global, u_command=global
  wires:
  deltas/1 -> Bus Selector/1
  Bus Selector/1 -> [delta_u]  "<delta_u>"
  Bus Selector/2 -> [delta_w]  "<delta_w>"
  Bus Selector/3 -> [delta_q]  "<delta_q>"
  Bus Selector/4 -> [delta_t]  "<delta_theta>"
  [delta_t] -> Radians to Degrees/1
  Radians to Degrees/1 -> To Workspace/1, Scope/1  "theta"
  [theta_command] -> To Workspace1/1, Scope/2  "theta_commanded"
  Subsystem/1(H) -> H/1  "H"
  Subsystem/3(alpha) -> Scope2/2  "alpha"
  Subsystem/2(gamma) -> Scope2/1  "gamma"
  Subsystem/4(theta) -> Scope2/3  "theta"
  Command/1 -> Bus Selector1/1
  Bus Selector1/1 -> [theta_command]  "<theta_command>"
  Bus Selector1/2 -> [u_command]  "<u_command>"
  [u_command] -> To Workspace3/1, u/2  "u_command"
  [delta_u] -> To Workspace2/1, u/1  "delat_u"
  Control_Actions/1 -> Bus Selector2/1
  Bus Selector2/1 -> Radians to Degrees1/1  "<delta_elevator>"
  Bus Selector2/2 -> Scope5/1  "<delta_thrust>"
  Radians to Degrees1/1 -> Scope4/1  "dlta_elevator"

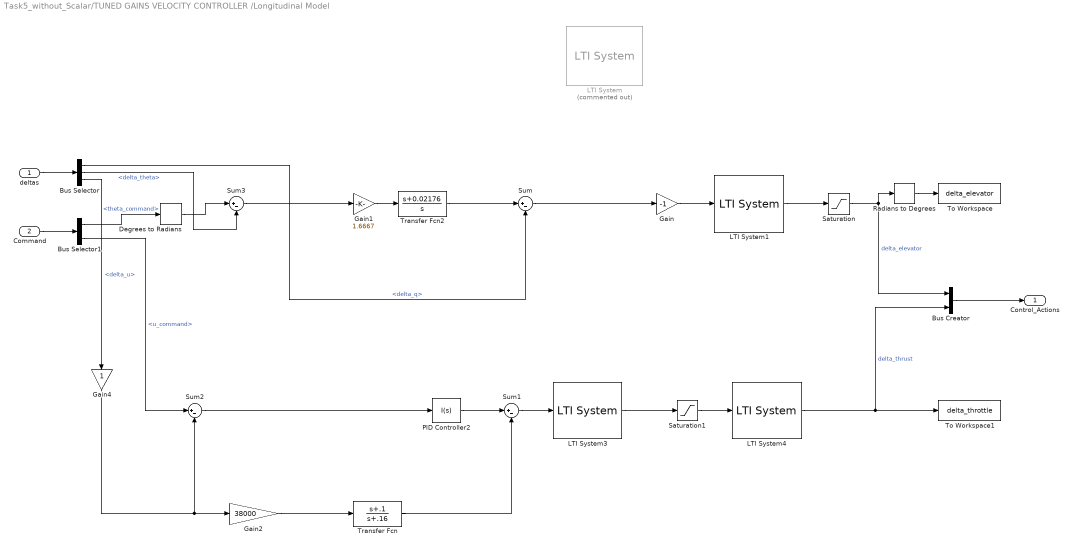
== system Task5_without_Scalar/TUNED GAINS VELOCITY CONTROLLER /Longitudinal Model ==
  deltas : Inport
  Command : Inport  Port=2
  Bus Creator : BusCreator  Inputs=2
  Bus Selector : BusSelector  OutputSignals=delta_q,delta_theta,delta_u
  Bus Selector1 : BusSelector  OutputSignals=theta_command,u_command
  Degrees to Radians : simulink_extras/Transformations/Degrees to Radians
  Gain : Gain  Gain=-1
  Gain1 : Gain  Gain=1.6667
  Gain2 : Gain  Gain=38000
  Gain4 : Gain
  LTI System : cstblocks/LTI System  Commented=on  sys=PI_Pitch  IC=[]  PadeOrder=0
  LTI System1 : cstblocks/LTI System  sys=servo  IC=[]  PadeOrder=0
  LTI System3 : cstblocks/LTI System  sys=servo  IC=[]  PadeOrder=0
  LTI System4 : cstblocks/LTI System  sys=Engine_Lag  IC=[]  PadeOrder=0
  PID Controller2 : slpidlib/PID Controller  Controller=I  Form=Parallel  TimeDomain=Continuous-time  UseExternalTs=off  SampleTime=-1  IntegratorMethod=Forward Euler  FilterMethod=Forward Euler  ControllerParametersSource=internal  P=25000  I=1400  UseKiTs=off  D=45918.9077381397  N=24.6739321802593  UseFilter=on  TunerSelectOption=Transfer Function Based (PID Tuner App)  InitialConditionSource=internal  InitialConditionForIntegrator=0  InitialConditionForFilter=0  DifferentiatorICPrevScaledInput=0  ExternalReset=none  TrackingMode=off  Kt=1  LimitOutput=off  SatLimitsSource=internal  UpperSaturationLimit=inf  LowerSaturationLimit=-inf  LinearizeAsGain=on  AntiWindupMode=none  Kb=1  LimitIntegrator=off  UpperIntegratorSaturationLimit=inf  LowerIntegratorSaturationLimit=-inf  POutMin=[]  POutMax=[]  IOutMin=[]  IOutMax=[]  DOutMin=[]  DOutMax=[]  NOutMin=[]  NOutMax=[]  SumOutMin=[]  SumOutMax=[]  SaturationOutMin=[]  SaturationOutMax=[]  PParamMin=[]  PParamMax=[]  IParamMin=[]  IParamMax=[]  DParamMin=[]  DParamMax=[]  NParamMin=[]  NParamMax=[]  KbParamMin=[]  KbParamMax=[]  KtParamMin=[]  KtParamMax=[]  KbOutMin=[]  KbOutMax=[]  KtOutMin=[]  KtOutMax=[]  IntegratorOutMin=[]  IntegratorOutMax=[]  FilterOutMin=[]  FilterOutMax=[]  SumI1OutMin=[]  SumI1OutMax=[]  SumI2OutMin=[]  SumI2OutMax=[]  SumI3OutMin=[]  SumI3OutMax=[]  SumI4OutMin=[]  SumI4OutMax=[]  SumDOutMin=[]  SumDOutMax=[]  DifferentiatorOutMin=[]  DifferentiatorOutMax=[]  FilterDiffOutCoefMin=[]  FilterDiffOutCoefMax=[]  ReciprocalOutMin=[]  ReciprocalOutMax=[]  SumDenOutMin=[]  SumDenOutMax=[]  SumNumOutMin=[]  SumNumOutMax=[]  DivideOutMin=[]  DivideOutMax=[]  UdiffTsProdOutMin=[]  UdiffTsProdOutMax=[]  NTsProdOutMin=[]  NTsProdOutMax=[]  UintegralTsProdOutMin=[]  UintegralTsProdOutMax=[]  UngainTsProdOutMin=[]  UngainTsProdOutMax=[]  ClampingZeroOutDataTypeStr=Inherit: Inherit via back propagation  ClampingZeroOutMin=[]  ClampingZeroOutMax=[]  FilterDenConstantOutDataTypeStr=Inherit: Inherit via back propagation  FilterDenConstantOutMin=[]  FilterDenConstantOutMax=[]  PCopyOutDataTypeStr=Inherit: Inherit via back propagation  PCopyOutMin=[]  PCopyOutMax=[]  NCopyOutDataTypeStr=Inherit: Inherit via back propagation  NCopyOutMin=[]  NCopyOutMax=[]  IntegratorContinuousStateAttributes=''  IntegratorStateMustResolveToSignalObject=off  IntegratorRTWStateStorageClass=Auto  FilterContinuousStateAttributes=''  FilterStateMustResolveToSignalObject=off  FilterRTWStateStorageClass=Auto  ParallelPVariant=Disabled  IdealPVariant=Disabled  IVariant=InternalParameters  DVariant=Disabled  IntegratorVariant=Continuous  SatVariant=Disabled  AWVariant=Passthrough  PCopyVariant=Disabled  TRVariant=Disabled  FdbkBlocksVariant=Forward  IdealPFdbkVariant=Disabled  SatFdbkVariant=Disabled  DerivativeFilterVariant=Disabled  NVariant=Disabled  NCopyVariant=Disabled_SignalSpec  FilterICVariant=Disabled  IntegratorICVariant=InternalICs  ExternalResetVariant=Disabled  TRSumVariant=Passthrough  SumFdbkVariant=Disabled  SumVariant=Passthrough_I  TsampFilterVariant=InternalTs  TsampNgainVariant=Passthrough  TsampIntegralVariant=Disabled_SignalSpec  ExternalSaturationOutDataTypeStr=Inherit: Same as second input
  Radians to Degrees : simulink_extras/Transformations/Radians to Degrees
  Saturation : Saturate  UpperLimit=deg2rad(25)  LowerLimit=deg2rad(-25)
  Saturation1 : Saturate  UpperLimit=65369  LowerLimit=-269369.84
  Sum{,1..3} (4 alike) : Sum  Inputs=|+-
  To Workspace : ToWorkspace  VariableName=delta_elevator  SampleTime=-1
  To Workspace1 : ToWorkspace  VariableName=delta_throttle  SampleTime=-1
  Transfer Fcn : TransferFcn  Numerator=[1 .1]  Denominator=[1 .16]
  Transfer Fcn2 : TransferFcn  Numerator=[1 0.02176]  Denominator=[1 0]
  Control_Actions : Outport
  wires:
  deltas/1 -> Bus Selector/1
  Command/1 -> Bus Selector1/1
  Bus Selector1/1 -> Degrees to Radians/1  "<theta_command>"
  Bus Selector/2 -> Sum3/2  "<delta_theta>"
  Degrees to Radians/1 -> Sum3/1
  Sum3/1 -> Gain1/1
  Bus Selector/1 -> Sum/2  "<delta_q>"
  Sum/1 -> Gain/1
  Gain/1 -> LTI System1/1
  LTI System1/1 -> Saturation/1
  Saturation/1 -> Bus Creator/1, Radians to Degrees/1  "delta_elevator"
  Bus Creator/1 -> Control_Actions/1
  Radians to Degrees/1 -> To Workspace/1
  Transfer Fcn2/1 -> Sum/1
  Bus Selector/3 -> Gain4/1  "<delta_u>"
  Sum2/1 -> PID Controller2/1
  Sum1/1 -> LTI System3/1
  LTI System3/1 -> Saturation1/1
  Saturation1/1 -> LTI System4/1
  Transfer Fcn/1 -> Sum1/2
  LTI System4/1 -> Bus Creator/2, To Workspace1/1  "delta_thrust"
  Bus Selector1/2 -> Sum2/1  "<u_command>"
  Gain1/1 -> Transfer Fcn2/1
  Gain4/1 -> Sum2/2, Gain2/1
  Gain2/1 -> Transfer Fcn/1
  PID Controller2/1 -> Sum1/1

== system Task5_without_Scalar/TUNED GAINS VELOCITY CONTROLLER /State Space Model ==
  Control_Actions : Inport
  Bus Creator1 : BusCreator  Inputs=4
  Bus Selector : BusSelector  OutputSignals=delta_elevator,delta_thrust
  Demux : Demux
  Gain : Gain  Gain=0
  Manual Switch : ManualSwitch
  Mux : Mux  Inputs=2
  State-Space : StateSpace  A=A_Long  B=B_Long  C=C_Long  D=D_Long  InitialCondition=0
  deltas : Outport
  wires:
  Demux/3 -> Bus Creator1/3  "delta_q"
  Mux/1 -> State-Space/1
  Demux/2 -> Bus Creator1/2  "delta_w"
  Demux/1 -> Bus Creator1/1  "delta_u"
  Bus Creator1/1 -> deltas/1
  State-Space/1 -> Demux/1
  Demux/4 -> Bus Creator1/4  "delta_theta"
  Manual Switch/1 -> Mux/2
  Gain/1 -> Manual Switch/2
  Control_Actions/1 -> Bus Selector/1
  Bus Selector/1 -> Mux/1  "<delta_elevator>"
  Bus Selector/2 -> Gain/1, Manual Switch/1  "<delta_thrust>"

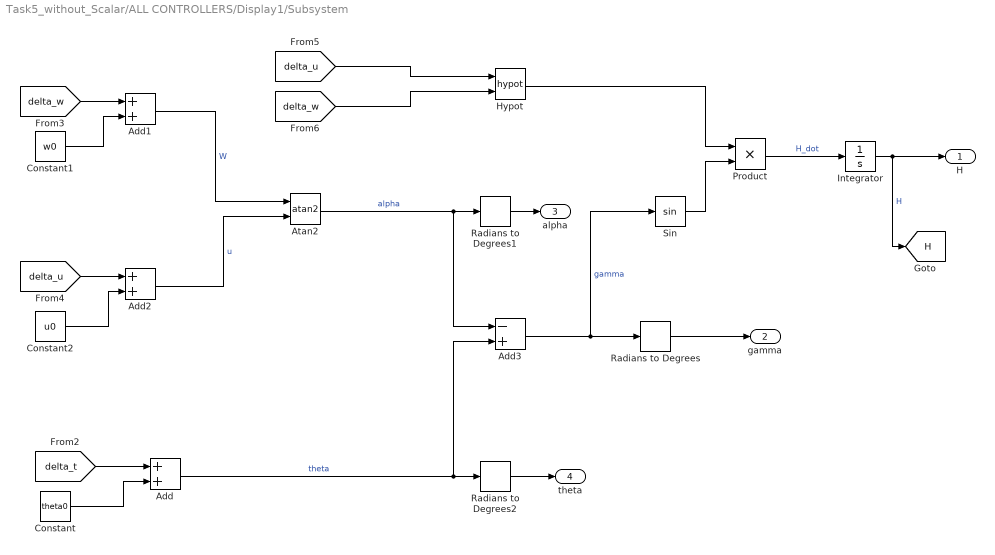
== system Task5_without_Scalar/ALL CONTROLLERS/Display1/Subsystem ==
  Add : Sum
  Add1 : Sum
  Add2 : Sum
  Add3 : Sum  Inputs=-+
  Atan2 : Trigonometry  Operator=atan2
  Constant : Constant  Value=theta0
  Constant1 : Constant  Value=w0
  Constant2 : Constant  Value=u0
  Hypot : Math  Operator=hypot
  Integrator : Integrator  InitialCondition=-states_0(12)
  Product : Product
  Radians to Degrees : simulink_extras/Transformations/Radians to Degrees
  Radians to Degrees1 : simulink_extras/Transformations/Radians to Degrees
  Radians to Degrees2 : simulink_extras/Transformations/Radians to Degrees
  Sin : Trigonometry
  H : Outport
  gamma : Outport  Port=2
  alpha : Outport  Port=3
  theta : Outport  Port=4
  tag scope: H=global
  wires:
  Radians to Degrees2/1 -> theta/1
  Radians to Degrees1/1 -> alpha/1
  Radians to Degrees/1 -> gamma/1
  Add1/1 -> Atan2/1  "W"
  Hypot/1 -> Product/1
  Atan2/1 -> Radians to Degrees1/1, Add3/1  "alpha"
  Add2/1 -> Atan2/2  "u"
  Product/1 -> Integrator/1  "H_dot"
  Add3/1 -> Sin/1, Radians to Degrees/1  "gamma"
  Constant/1 -> Add/2
  Constant2/1 -> Add2/2
  [delta_w] -> Add1/1
  [delta_u] -> Add2/1
  Sin/1 -> Product/2
  Constant1/1 -> Add1/2
  [delta_u] -> Hypot/1
  Add/1 -> Add3/2, Radians to Degrees2/1  "theta"
  [delta_t] -> Add/1
  Integrator/1 -> [H], H/1  "H"
  [delta_w] -> Hypot/2

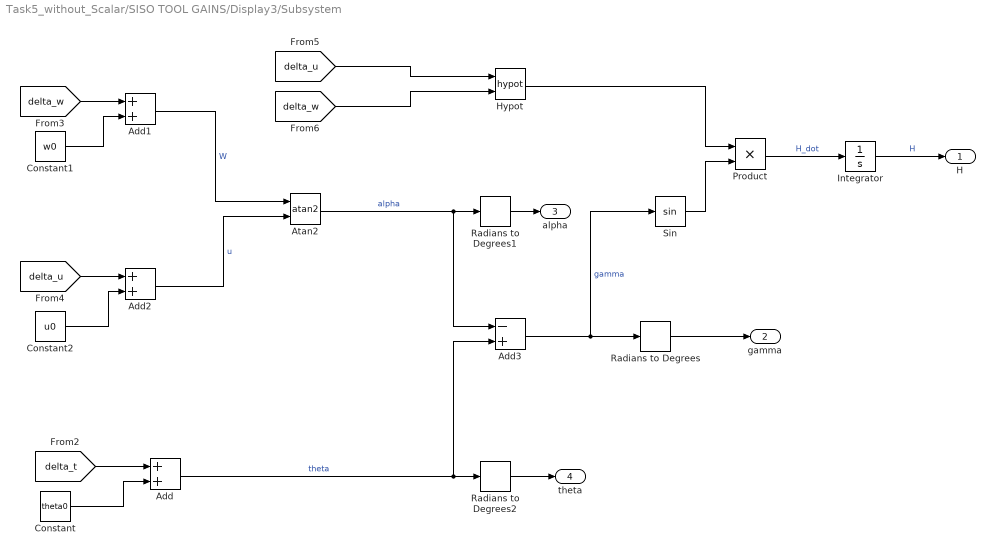
== system Task5_without_Scalar/SISO TOOL GAINS/Display3/Subsystem ==
  Add : Sum
  Add1 : Sum
  Add2 : Sum
  Add3 : Sum  Inputs=-+
  Atan2 : Trigonometry  Operator=atan2
  Constant : Constant  Value=theta0
  Constant1 : Constant  Value=w0
  Constant2 : Constant  Value=u0
  Hypot : Math  Operator=hypot
  Integrator : Integrator  InitialCondition=-states_0(12)
  Product : Product
  Radians to Degrees : simulink_extras/Transformations/Radians to Degrees
  Radians to Degrees1 : simulink_extras/Transformations/Radians to Degrees
  Radians to Degrees2 : simulink_extras/Transformations/Radians to Degrees
  Sin : Trigonometry
  H : Outport
  gamma : Outport  Port=2
  alpha : Outport  Port=3
  theta : Outport  Port=4
  wires:
  [delta_w] -> Hypot/2
  Integrator/1 -> H/1  "H"
  [delta_t] -> Add/1
  Add/1 -> Radians to Degrees2/1, Add3/2  "theta"
  [delta_u] -> Hypot/1
  Constant1/1 -> Add1/2
  Sin/1 -> Product/2
  [delta_u] -> Add2/1
  [delta_w] -> Add1/1
  Constant2/1 -> Add2/2
  Constant/1 -> Add/2
  Add3/1 -> Radians to Degrees/1, Sin/1  "gamma"
  Product/1 -> Integrator/1  "H_dot"
  Add2/1 -> Atan2/2  "u"
  Atan2/1 -> Add3/1, Radians to Degrees1/1  "alpha"
  Hypot/1 -> Product/1
  Add1/1 -> Atan2/1  "W"
  Radians to Degrees/1 -> gamma/1
  Radians to Degrees1/1 -> alpha/1
  Radians to Degrees2/1 -> theta/1

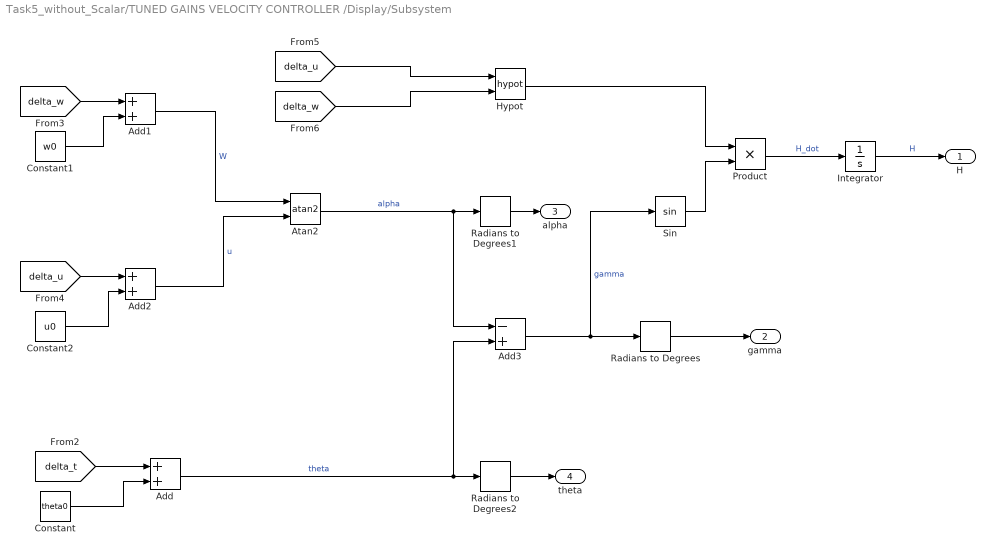
== system Task5_without_Scalar/TUNED GAINS VELOCITY CONTROLLER /Display/Subsystem ==
  Add : Sum
  Add1 : Sum
  Add2 : Sum
  Add3 : Sum  Inputs=-+
  Atan2 : Trigonometry  Operator=atan2
  Constant : Constant  Value=theta0
  Constant1 : Constant  Value=w0
  Constant2 : Constant  Value=u0
  Hypot : Math  Operator=hypot
  Integrator : Integrator  InitialCondition=-states_0(12)
  Product : Product
  Radians to Degrees : simulink_extras/Transformations/Radians to Degrees
  Radians to Degrees1 : simulink_extras/Transformations/Radians to Degrees
  Radians to Degrees2 : simulink_extras/Transformations/Radians to Degrees
  Sin : Trigonometry
  H : Outport
  gamma : Outport  Port=2
  alpha : Outport  Port=3
  theta : Outport  Port=4
  wires:
  [delta_w] -> Hypot/2
  Integrator/1 -> H/1  "H"
  [delta_t] -> Add/1
  Add/1 -> Radians to Degrees2/1, Add3/2  "theta"
  [delta_u] -> Hypot/1
  Constant1/1 -> Add1/2
  Sin/1 -> Product/2
  [delta_u] -> Add2/1
  [delta_w] -> Add1/1
  Constant2/1 -> Add2/2
  Constant/1 -> Add/2
  Add3/1 -> Radians to Degrees/1, Sin/1  "gamma"
  Product/1 -> Integrator/1  "H_dot"
  Add2/1 -> Atan2/2  "u"
  Atan2/1 -> Add3/1, Radians to Degrees1/1  "alpha"
  Hypot/1 -> Product/1
  Add1/1 -> Atan2/1  "W"
  Radians to Degrees/1 -> gamma/1
  Radians to Degrees1/1 -> alpha/1
  Radians to Degrees2/1 -> theta/1
